simulink model "servo2"  (Simulink 8.1)
settings: Solver=ode45  StartTime=0.0  StopTime=10.0  RelTol=1e-3
undefined symbols (not defined in the file or in its folder): Kv
settings Model: Creator=mainster  LastModifiedBy=mainster
settings OptimizationCC: BlockReduction=off  BooleanDataType=off  ExpressionDepthLimit=128
settings DebuggingCC: SaveWithParameterizedLinksMsg=none  SignalResolutionControl=TryResolveAllWithWarning  SolverPrmCheckMsg=none  MultiTaskDSMMsg=warning  MultiTaskCondExecSysMsg=none  FcnCallInpInsideContextMsg=EnableAllAsError  StrictBusMsg=None
settings HardwareCC: TargetUnknown=on
settings RTWCC: IncludeERTFirstTime=on

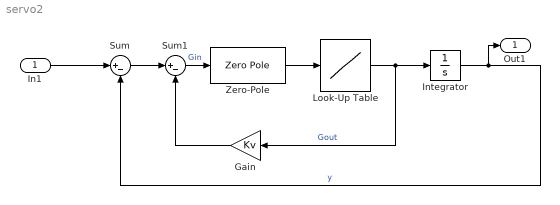
== system servo2 ==
  In1 : Inport
  Gain : Gain  Gain=Kv  SaturateOnIntegerOverflow=on  OutDataTypeStr=Inherit: Same as input  ParamDataTypeStr=Inherit: Same as input
  Integrator : Integrator
  Look-Up Table : Lookup  InputValues=[-5:5]  Table=tanh([-5:5])*2  SaturateOnIntegerOverflow=on
  Sum : Sum  Inputs=|+-  SaturateOnIntegerOverflow=on  InputSameDT=on  OutDataTypeStr=Inherit: Same as first input
  Sum1 : Sum  Inputs=|+-  SaturateOnIntegerOverflow=on  InputSameDT=on  OutDataTypeStr=Inherit: Same as first input
  Zero-Pole : ZeroPole  Zeros=[ ]  Poles=[-5 -1]  Gain=[5]
  Out1 : Outport
  wires:
  Sum/1 -> Sum1/1
  Sum1/1 -> Zero-Pole/1  "Gin"
  Zero-Pole/1 -> Look-Up Table/1
  Gain/1 -> Sum1/2
  Look-Up Table/1 -> Gain/1, Integrator/1  "Gout"
  Integrator/1 -> Out1/1, Sum/2  "y"
  In1/1 -> Sum/1
